simulink model "transformer_model_latest"  (Simulink 8.1)
settings: Solver=ode45  StartTime=0.0  StopTime=2  RelTol=1e-3
undefined symbols (not defined in the file or in its folder): D1, Delta
libraries: powerlib x9
settings Model: Creator=MihnathulMunthaha  LastModifiedBy=root
settings DataIOCC: SignalLoggingSaveFormat=Dataset
settings DebuggingCC: FcnCallInpInsideContextMsg=EnableAllAsError
settings GRTTargetCC: CombineOutputUpdateFcns=on  GRTInterface=off

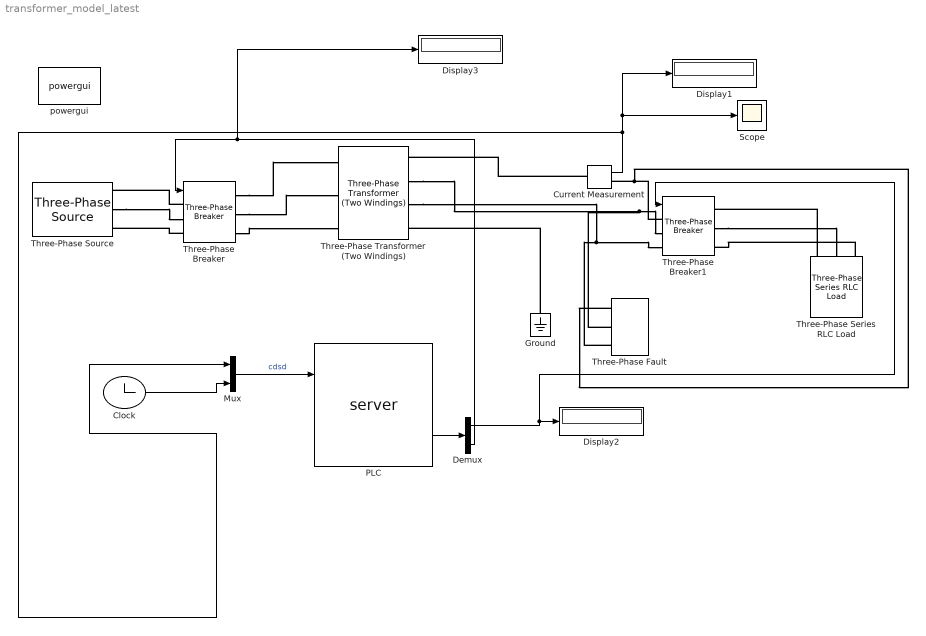
== system transformer_model_latest ==
  Clock : Clock
  Current Measurement : powerlib/Measurements/Current Measurement  PhasorSimulation=off  OutputType=Complex  PSBequivalent=0
  Demux : Demux  Outputs=2
  Display1 : Display
  Display2 : Display
  Display3 : Display
  Ground : powerlib/Elements/Ground  LConnTagsString=a
  Mux : Mux  Inputs=2
  PLC : S-Function  Priority=1  FunctionName=server  Parameters=portNumber, optionProtocole, optionEndian  EnableBusSupport=off  mask(Server){portNumber=502, optionProtocole=TCP, optionEndian=Big Endian}
      mask prompts: portNumber "Number of port"; optionProtocole "Protocole"; optionEndian "Endianess"
      mask TypeOptions optionProtocole: TCP | UDP
      mask TypeOptions optionEndian: Big Endian | Little Endian
      mask Display:
      | image(imread('PLC.jpg'))
      | port_label('input', 1, 'AI');
      | port_label('input', 2, 'DI');
      | port_label('output', 1, 'AO');
      | port_label('output', 2, 'DO');
  Scope : Scope
      settings: TimeRange=0.2  YMin=-550  YMax=350  MaxDataPoints=5000000
  Three-Phase Breaker : powerlib/Elements/Three-Phase Breaker  InitialState=closed  SwitchA=on  SwitchB=on  SwitchC=on  SwitchTimes="[1/60  2/60]"  External=on  BreakerResistance=0.001  SnubberResistance=1e6  SnubberCapacitance=inf  Measurements=Breaker currents
  Three-Phase Breaker1 : powerlib/Elements/Three-Phase Breaker  InitialState=closed  SwitchA=on  SwitchB=on  SwitchC=on  SwitchTimes="[4/60  10/60]"  External=on  BreakerResistance=0.001  SnubberResistance=1e6  SnubberCapacitance=inf  Measurements=Breaker currents
  Three-Phase Fault : powerlib/Elements/Three-Phase Fault  FaultA=on  FaultB=on  FaultC=on  FaultResistance=0.00001  GroundFault=on  GroundResistance=0.001  External=off  SwitchStatus=[1 0]  SwitchTimes=[ 0.03 0.0496]  InitialStates=[0 0 1]  SnubberResistance=1e6  SnubberCapacitance=inf  Measurements=None
  Three-Phase Series RLC Load : powerlib/Elements/Three-Phase Series RLC Load  LConnTagsString=A|B|C  Configuration=Y (grounded)  NominalVoltage=315e3  NominalFrequency=180  ActivePower=250e6  InductivePower=0  CapacitivePower=0  Measurements=None  LoadType=constant Z
  Three-Phase Source : powerlib/Electrical Sources/Three-Phase Source  Voltage=735e3  PhaseAngle=0  Frequency=180  InternalConnection=Yn  SpecifyImpedance=on  Resistance=0.8929  Inductance=16.58e-3  ShortCircuitLevel=250e6  BaseVoltage=735e3  XRratio=7  BusType=swing  Pref=0  Qref=0  Qmin=-inf  Qmax=inf
  Three-Phase Transformer (Two Windings) : powerlib/Elements/Three-Phase Transformer (Two Windings)  Winding1Connection=Delta (D1)  UNITS=SI  NominalPower=[ 250e6 ,180 ]  Winding1=[7.35e+05 12.965 1.3757]  Winding2Connection=Yn  Winding2=[3.15e+05 0.7938 0.084225]  SetSaturation=off  Rm=3.2414e+06  Lm=8597.9  Saturation=[0 0;0.38482 3308.7;160.34 4191]  Hysteresis=off  DataFile='hysteresis'  SetInitialFlux=off  InitialFluxes=[2205.8 -2205.8 1930.1]  Measurements=None  MoreParameters=off  BreakLoop=off  DataType=on  TransfoNumber=1
  powergui : powerlib/powergui  Priority=1  SimulationMode=Continuous  SolverType=Tustin  SampleTime=50e-6  frequency=60  SPID=off  DisableSnubberDevices=off  DisableRonSwitches=off  DisableVfSwitches=off  SwTol=0  Interpol=off  DisplayEquations=off  frequencyindice=0  Pbase=100e6  ErrMax=1e-4  Iterations=50  UnitsV=kV  UnitsW=MW  FunctionMessages=on  echomessages=off  HookPort=off  EnableUseOfTLC=off  x0status=blocks  RestoreLinks=warning  ResistiveCurrentMeasurement=off  Frange=[0:2:500]  Ylog=off  Xlog=off  ShowGrid=on  save=off  variable=ZData  ZoomFFT=off  StartTime=0.0  cycles=1  DisplayStyle=1  fundamental=60  FreqAxis=off  MaxFrequency=1000  frequencyindicesteady=1  RmsSteady=1  display=off  Ts=0  methode=off
  wires:
  Current Measurement/1 -> Mux/1, Display1/1, Scope/1
  Mux/1 -> PLC/1  "cdsd"
  Clock/1 -> Mux/2
  PLC/2 -> Demux/1
  Demux/2 -> Display3/1, Three-Phase Breaker/1
  Demux/1 -> Three-Phase Breaker1/1, Display2/1
  connections:
  Ground/LConn1 -- Three-Phase Transformer (Two Windings)/RConn4
  Current Measurement/LConn1 -- Three-Phase Transformer (Two Windings)/RConn1
  Three-Phase Breaker/LConn1 -- Three-Phase Source/RConn1
  Three-Phase Breaker/RConn3 -- Three-Phase Transformer (Two Windings)/LConn3
  Three-Phase Breaker/RConn2 -- Three-Phase Transformer (Two Windings)/LConn2
  Three-Phase Source/RConn2 -- Three-Phase Breaker/LConn2
  Three-Phase Breaker/LConn3 -- Three-Phase Source/RConn3
  Three-Phase Breaker1/LConn1 -- Three-Phase Fault/LConn1 -- Current Measurement/RConn1
  Three-Phase Transformer (Two Windings)/RConn2 -- Three-Phase Fault/LConn2 -- Three-Phase Breaker1/LConn2
  Three-Phase Transformer (Two Windings)/RConn3 -- Three-Phase Breaker1/LConn3 -- Three-Phase Fault/LConn3
  Three-Phase Series RLC Load/LConn1 -- Three-Phase Breaker1/RConn1
  Three-Phase Breaker1/RConn2 -- Three-Phase Series RLC Load/LConn2
  Three-Phase Series RLC Load/LConn3 -- Three-Phase Breaker1/RConn3
  Three-Phase Breaker/RConn1 -- Three-Phase Transformer (Two Windings)/LConn1
